simulink model "WT"  (R2016a)
settings: Solver=VariableStepAuto  StartTime=0.0  StopTime=10.0  RelTol=1e-3
settings Model: Creator=cinlab  LastModifiedBy=cinlab

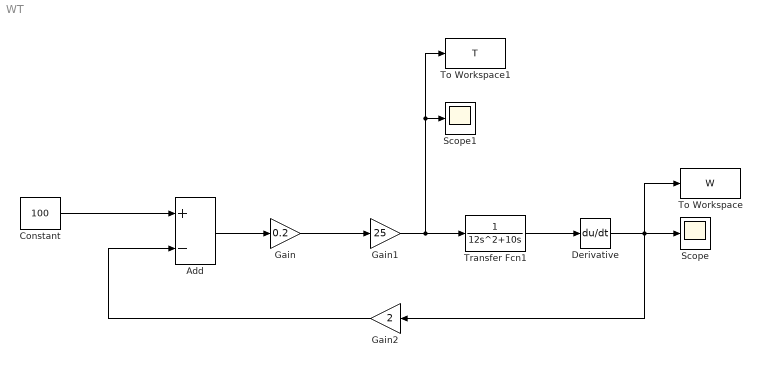
== system WT ==
  Add : Sum  Inputs=+-
  Constant : Constant  Value=100
  Derivative : Derivative
  Gain : Gain  Gain=0.2
  Gain1 : Gain  Gain=25
  Gain2 : Gain  Gain=2
  Scope : Scope
  Scope1 : Scope
  To Workspace : ToWorkspace  VariableName=W  SampleTime=-1
  To Workspace1 : ToWorkspace  VariableName=T  SampleTime=-1
  Transfer Fcn1 : TransferFcn  Denominator=[12 10 0]
  wires:
  Constant/1 -> Add/1
  Gain/1 -> Gain1/1
  Gain1/1 -> To Workspace1/1, Scope1/1, Transfer Fcn1/1
  Add/1 -> Gain/1
  Transfer Fcn1/1 -> Derivative/1
  Derivative/1 -> To Workspace/1, Gain2/1, Scope/1
  Gain2/1 -> Add/2
